simulink model "antilock_braking_system"  (R2020b)
settings: Solver=VariableStepAuto  StartTime=0.0  StopTime=10.0  RelTol=1e-3
values from neighbouring files (symbols this model uses):
  I = 5    [data.m]    (also in sldemo_absdata.m)
  Kf = 1    [data.m]    (also in sldemo_absdata.m)
  PBmax = 1500    [data.m]    (also in sldemo_absdata.m)
  Rr = 15/12    (= 1.25)    [data.m]    (also in sldemo_absdata.m)
  v0 = 88    [data.m]    (also in sldemo_absdata.m)
settings Model: Creator=WELCOME  LastModifiedBy=WELCOME

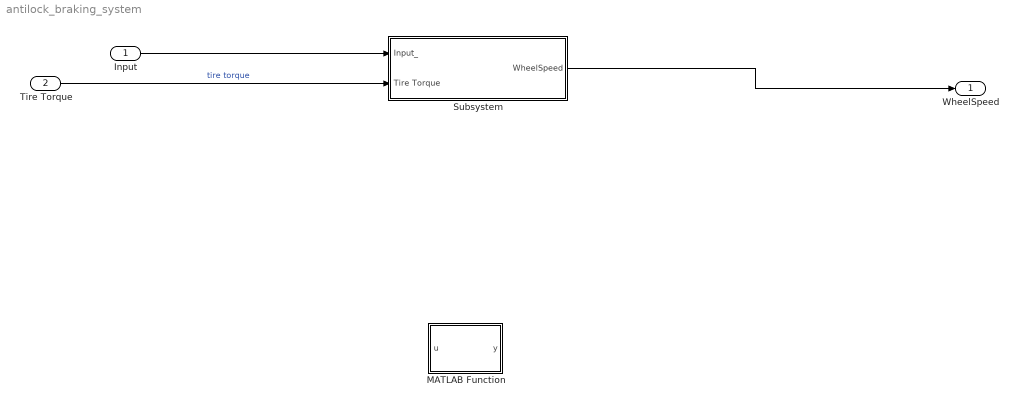
== system antilock_braking_system ==
  Input : Inport  SampleTime=0
  Tire Torque : Inport  Port=2
  MATLAB Function : MATLAB Function  TreatAsAtomicUnit=on
  Subsystem : Subsystem
  WheelSpeed : Outport  VectorParamsAs1DForOutWhenUnconnected=off
  wires:
  Input/1 -> Subsystem/1(Input_)
  Tire Torque/1 -> Subsystem/2(Tire Torque)  "tire torque"
  Subsystem/1(WheelSpeed) -> WheelSpeed/1

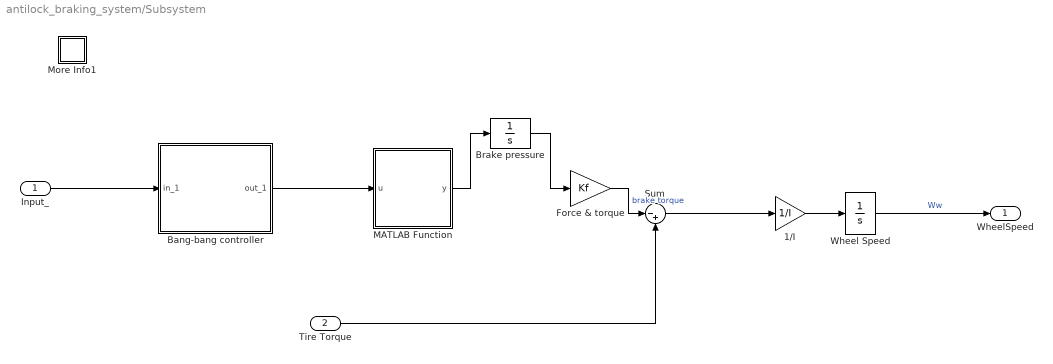
== system antilock_braking_system/Subsystem ==
  Input_ : Inport  SampleTime=0
  Tire Torque : Inport  Port=2
  1/I : Gain  Gain=1/I  SaturateOnIntegerOverflow=on  OutDataTypeStr=Inherit: Same as input  ParamDataTypeStr=Inherit: Same as input
  Bang-bang controller : Subsystem  mask(Sign){}
      mask help: y = sign(x)
      mask Help: Sign Function:\n\t\t\ty = 1 if x > 0\n\t\t\ty = 0 if x = 0\n\t\t\ty = -1 if x < 0
      mask Display: plot(-50,-50,50,50,[-50,50],[0,0],[0,0],[-50,50],[-40,0],[-30,-30],[0,40],[30,30])
  Brake pressure : Integrator  LimitOutput=on  UpperSaturationLimit=PBmax  LowerSaturationLimit=0
  Force & torque : Gain  Gain=Kf  SaturateOnIntegerOverflow=on  OutDataTypeStr=Inherit: Same as input  ParamDataTypeStr=Inherit: Same as input
  MATLAB Function : MATLAB Function  TreatAsAtomicUnit=on
  More Info1 : Subsystem
      settings: OpenFcn=showExample('simulink_automotive/ModelingAnAntiLockBrakingSystemExample')
      mask Display: disp('?')
  Sum : Sum  Inputs=|-+  InputSameDT=on  SaturateOnIntegerOverflow=on  OutDataTypeStr=Inherit: Same as first input
  Wheel Speed : Integrator  InitialCondition=v0/Rr  LimitOutput=on  UpperSaturationLimit=1000  LowerSaturationLimit=0
  WheelSpeed : Outport  VectorParamsAs1DForOutWhenUnconnected=off
  wires:
  Sum/1 -> 1/I/1
  Bang-bang controller/1(out_1) -> MATLAB Function/1(u)
  Input_/1 -> Bang-bang controller/1(in_1)
  Wheel Speed/1 -> WheelSpeed/1  "Ww"
  1/I/1 -> Wheel Speed/1
  MATLAB Function/1(y) -> Brake pressure/1
  Force & torque/1 -> Sum/1  "brake torque"
  Tire Torque/1 -> Sum/2
  Brake pressure/1 -> Force & torque/1

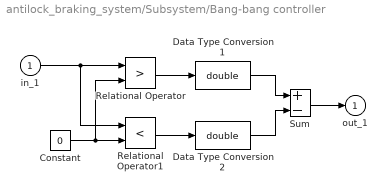
== system antilock_braking_system/Subsystem/Bang-bang controller ==
  in_1 : Inport
  Constant : Constant  Value=0
  Data Type Conversion1 : DataTypeConversion  OutDataTypeStr=double  SaturateOnIntegerOverflow=on  RndMeth=Zero
  Data Type Conversion2 : DataTypeConversion  OutDataTypeStr=double  SaturateOnIntegerOverflow=on  RndMeth=Zero
  Relational Operator : RelationalOperator  Operator=>  OutDataTypeStr=boolean  RndMeth=Nearest  InputSameDT=on
  Relational Operator1 : RelationalOperator  Operator=<  OutDataTypeStr=boolean  RndMeth=Nearest  InputSameDT=on
  Sum : Sum  Inputs=+-  InputSameDT=on  SaturateOnIntegerOverflow=on  OutDataTypeStr=Inherit: Same as first input
  out_1 : Outport  InitialOutput=0  VectorParamsAs1DForOutWhenUnconnected=off
  wires:
  Data Type Conversion2/1 -> Sum/2
  Data Type Conversion1/1 -> Sum/1
  Sum/1 -> out_1/1
  Relational Operator/1 -> Data Type Conversion1/1
  Relational Operator1/1 -> Data Type Conversion2/1
  Constant/1 -> Relational Operator/2, Relational Operator1/2
  in_1/1 -> Relational Operator1/1, Relational Operator/1

== system antilock_braking_system/Subsystem/More Info1 ==

== matlab function antilock_braking_system/Subsystem/MATLAB Function ==
  data: u input; y output
function y = fcn(u)

y =100 u/(TB+1);

== matlab function antilock_braking_system/MATLAB Function ==
  data: u input; y output
function y = fcn(u)

y = 1.0 - u(1)/(u(2) + (u(2)==0)*eps);
